simulink model "Series_R2015b"  (R2017a)
settings: Solver=ode4  StartTime=0  StopTime=1200  FixedStep=0.1  MaxStep=0.05  RelTol=1e-5
values from neighbouring files (symbols this model uses):
  Av = 2.289    [Plan_Series_initiate.m]    (also in Series_initiate.m = 2.57025)
  Cd = 0.254    [Plan_Series_initiate.m]    (also in Series_initiate.m = 0.26)
  Cr = 0.008    [Plan_Series_initiate.m]    (also in Series_initiate.m)
  Density = 32e6    (= 32000000)    [Plan_Series_initiate.m]    (also in Series_initiate.m = 21460000)
  EtaEM1 = [0.01 0.01 0.01 0.01 0.01 0.01 0.01 0.01 0.01 0.01 0.01 0.01 ... (294 elements, 14x21)]    [EtaEM_THS.mat]
  EtaEM2 = [0.01 0.85 0.85 0.85 0.8 0.8 0.75 0.7 0.7 0.65 0.65 0.6 ... (234 elements, 18x13)]    [EtaEM_THS.mat]
  EtaPE = .98    (= 0.98)    [Plan_Series_initiate.m]    (also in Series_initiate.m)
  gr2 = 5    [Plan_Series_initiate.m]    (also in Series_initiate.m)
  grav = 9.81    [Plan_Series_initiate.m]    (also in Series_initiate.m)
  Jgenset = 0.15    [Plan_Series_initiate.m]    (also in Series_initiate.m = 0.1)
  kgenset = Jgenset/4/0.05    (= 0.5)    [Series_initiate.m]
  ksoc = Wbatt/400/Tau_charge    (= 1179.36)    [Plan_Series_initiate.m]    (also in Series_initiate.m = 11700)
  Mv = 1300    [Plan_Series_initiate.m]    (also in Series_initiate.m = 1575)
  OnOffMax = SOC_batt_ref_value-eps    [Plan_Series_initiate.m]    (also in Series_initiate.m)
  OnOffMin = 30    [Plan_Series_initiate.m]    (also in Series_initiate.m)
  Paux = 600    [Plan_Series_initiate.m]    (also in Series_initiate.m)
  Pice_max = wice_max*Tice_max    (= 49480.084294)    [Plan_Series_initiate.m]    (also in Series_initiate.m = 5000)
  PtoT = zeros(length(P),4)    [CreateICEmap.m]
  rho_air = 1.225    [Plan_Series_initiate.m]    (also in Series_initiate.m)
  rw = 0.301    [Plan_Series_initiate.m]    (also in Series_initiate.m = 0.3)
  SOC_batt_ref_value = 70    [Plan_Series_initiate.m]    (also in Series_initiate.m)
  Tau_charge = 10    [Plan_Series_initiate.m]    (also in Series_initiate.m = 1)
  Tem1_max = 31    [Plan_Series_initiate.m]    (also in Series_initiate.m = 1.2*Tice_max)
  Tem2_max = 400    [Plan_Series_initiate.m]    (also in Series_initiate.m = 200)
  Tice_max = 105    [Plan_Series_initiate.m]    (also in Series_initiate.m = Pice_max/(wice_max*row/(length(EtaICE)-1)))
  Wbatt = 201.6*6.5*3600    (= 4717440)    [Plan_Series_initiate.m]    (also in Series_initiate.m = 4680000)
  wice_max = 4500*2*pi/60    (= 471.238898038)    [Plan_Series_initiate.m]    (also in Series_initiate.m)
  wice_min = 1000*2*pi/60    (= 104.71975512)    [Plan_Series_initiate.m]    (also in Series_initiate.m = 83.7758040957)
undefined symbols (not defined in the file or in its folder): EtaBATT, Pbatt, Pice_max_parallel, sfunxy, Tlim_ice, Wice
undefined symbols (not defined in the file): EtaICE, FuelConsICE, Pem1_max, Pem2_max, Tem1, Tem2, Tice, Wem1, Wem2
(part 2 of 2)

== system Series_R2015b/ICE-model/wt (ICE) ==
  x : Inport
  y : Inport  Port=2
  Mux : Mux  Inputs=2
  sfunxy : S-Function  DisableCoverage=on  FunctionName=sfunxy  Parameters=[xmin xmax ymin ymax], st  SFunctionDeploymentMode=off  EnableBusSupport=off
  wires:
  y/1 -> Mux/2
  x/1 -> Mux/1
  Mux/1 -> sfunxy/1

== system Series_R2015b/Control of the drivetrain/Optimal operating point for ICE (figure 11)/Low pass -filter for dynamic limitation (page 18) ==
  P chargemom : Inport
  Gain2 : Gain  Gain=1/(Tau_charge)  SaturateOnIntegerOverflow=on  OutDataTypeStr=Inherit: Same as input  ParamDataTypeStr=Inherit: Same as input
  Sum3 : Sum  Inputs=+-  SaturateOnIntegerOverflow=on  InputSameDT=on  OutDataTypeStr=Inherit: Same as first input
  Wbatt : Integrator  UpperSaturationLimit=Pice_max_parallel  LowerSaturationLimit=0
  P charge * : Outport  InitialOutput=0
  wires:
  P chargemom/1 -> Sum3/1
  Sum3/1 -> Gain2/1
  Gain2/1 -> Wbatt/1
  Wbatt/1 -> Sum3/2, P charge */1
